simulink model "diffcar"  (Simulink 9.3)
settings: Solver=ode45  StartTime=0.0  StopTime=10  RelTol=1e-3  EnableMultiTasking=on
libraries: simulink x1
settings Model: Creator=Gu  LastModifiedBy=gufang
settings DataIOCC: LimitDataPoints=on
settings OptimizationCC: ExpressionDepthLimit=2147483647
settings DebuggingCC: SolverPrmCheckMsg=warning  StateNameClashWarn=warning  SFExecutionAtInitializationDiag=warning
settings SFSimCC: SimParseCustomCode=off
settings GRTTargetCC: GeneratePreprocessorConditionals=Disable all
settings ConfigComp: CovSFcnEnable=off

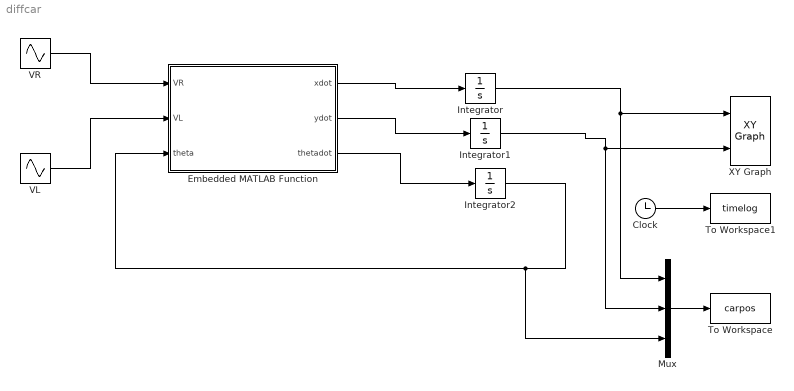
== system diffcar ==
  Clock : Clock
  Embedded MATLAB Function : MATLAB Function  TreatAsAtomicUnit=on
  Integrator : Integrator
  Integrator1 : Integrator
  Integrator2 : Integrator
  Mux : Mux  Inputs=3
  To Workspace : ToWorkspace  VariableName=carpos  SampleTime=0.05
  To Workspace1 : ToWorkspace  VariableName=timelog  SampleTime=-1
      settings: Save2DSignal=2-D array (concatenate along first dimension)
  VL : Sin  Frequency=0.2  SampleTime=0
  VR : Sin  Frequency=0.5  SampleTime=0
  XY Graph : simulink/Sinks/XY Graph  xmin=-10  xmax=10  ymin=-10  ymax=10  st=-1
  wires:
  VR/1 -> Embedded MATLAB Function/1(VR)
  VL/1 -> Embedded MATLAB Function/2(VL)
  Embedded MATLAB Function/1(xdot) -> Integrator/1
  Embedded MATLAB Function/2(ydot) -> Integrator1/1
  Embedded MATLAB Function/3(thetadot) -> Integrator2/1
  Integrator2/1 -> Embedded MATLAB Function/3(theta), Mux/3
  Integrator/1 -> XY Graph/1, Mux/1
  Integrator1/1 -> XY Graph/2, Mux/2
  Mux/1 -> To Workspace/1
  Clock/1 -> To Workspace1/1

== matlab function Embedded MATLAB Function ==
  data: VR input double; xdot output double; VL input double; theta input double; ydot output double; thetadot output double
function [xdot, ydot, thetadot] = fcn(VR, VL,theta)

d=0.5; % axial space
xdot=(VR+VL)/2*cos(theta);
ydot=(VR+VL)/2*sin(theta);
thetadot=(VR-VL)/d;
